simulink model "off_sentric_disc"  (R2020a)
settings: Solver=VariableStepAuto  StartTime=0.0  StopTime=10.0  RelTol=1e-3
values from neighbouring files (symbols this model uses):
  g = @(t)    [boat_riccati.m]    (also in butterfly_robot.m = [g_w;g_y_dot;g_y]; butterfly_robot_phi_varphi.m = [g_w;g_y_dot;g_y]; homework_5.m = 9.81; test_drawing.m = hgtransform)
  phi = q(2)    [butterfly_robot.m]    (also in jalla_lqr.m = atan2(y_dot,x_dot); plot_all_functions.m = linspace(0,2*pi,1000); plotting_phi_varphi.m = linspace(0,2*pi,1000); test_lmi.m = linspace(0,pi,N))
  psi = @(t) omega_c*t+psi_0    [boat_riccati.m]    (also in homework_5.m = @(x,y) (cos(y+m_g(x))^2-2)/(cos(y+m_g(x))+der_m_g(x)); jalla_lqr.m = atan2(y, x))
undefined symbols (not defined in the file or in its folder): m, mu, rcm, xcb, ycb
settings Model: Creator=g-oft  LastModifiedBy=g-oft

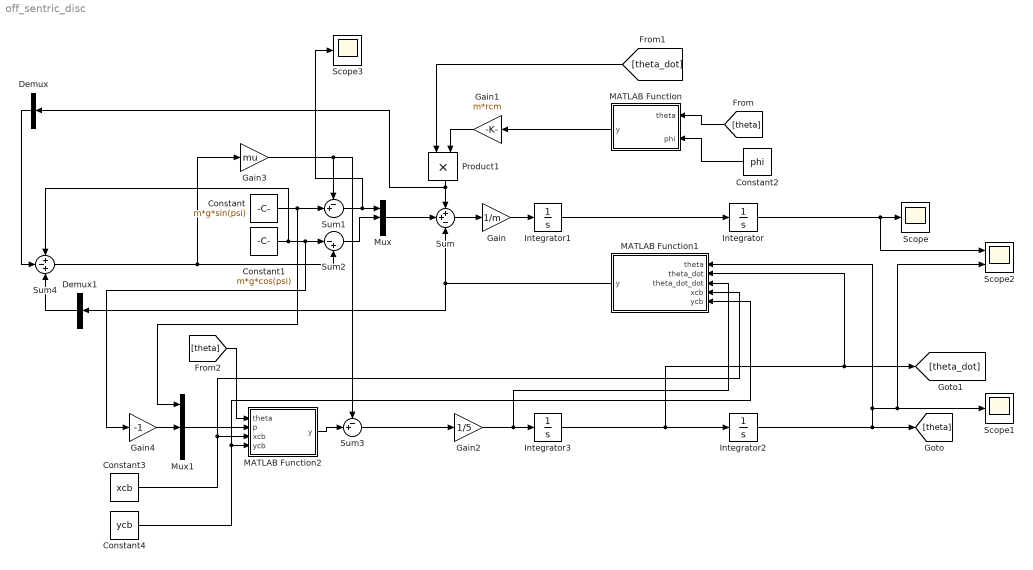
== system off_sentric_disc ==
  Constant : Constant  Value=m*g*sin(psi)
  Constant1 : Constant  Value=m*g*cos(psi)
  Constant2 : Constant  Value=phi
  Constant3 : Constant  Value=xcb
  Constant4 : Constant  Value=ycb
  Demux : Demux  Outputs=3
  Demux1 : Demux  Outputs=3
  Gain : Gain  Gain=1/m
  Gain1 : Gain  Gain=m*rcm
  Gain2 : Gain  Gain=1/5
  Gain3 : Gain  Gain=mu
  Gain4 : Gain  Gain=-1
  Integrator{,1..3} (4 alike) : Integrator
  MATLAB Function : MATLAB Function  TreatAsAtomicUnit=on
  MATLAB Function1 : MATLAB Function  TreatAsAtomicUnit=on
  MATLAB Function2 : MATLAB Function  TreatAsAtomicUnit=on
  Mux : Mux  Inputs=3
  Mux1 : Mux  Inputs=3
  Product1 : Product
  Scope : Scope
  Scope1 : Scope
  Scope2 : Scope  NumInputPorts=2
  Scope3 : Scope
  Sum : Sum  Inputs=++-
  Sum1 : Sum  Inputs=-+|
  Sum2 : Sum  Inputs=|-+
  Sum3 : Sum  Inputs=-+|
  Sum4 : Sum  Inputs=+-+
  wires:
  Integrator1/1 -> Integrator/1
  Integrator3/1 -> MATLAB Function1/2(theta_dot), [theta_dot], Integrator2/1
  Constant/1 -> Mux1/1, Sum1/2
  Sum1/1 -> Scope3/1, Mux/1
  Constant1/1 -> Gain4/1, Sum2/1, Sum4/1
  Sum2/1 -> Mux/2
  Mux/1 -> Sum/2
  Sum/1 -> Gain/1
  Gain/1 -> Integrator1/1
  [theta] -> MATLAB Function/1(theta)
  Integrator2/1 -> MATLAB Function1/1(theta), Scope2/2, Scope1/1, [theta]
  MATLAB Function/1(y) -> Gain1/1
  Product1/1 -> Demux/1, Sum/1
  Gain1/1 -> Product1/2
  [theta_dot] -> Product1/1
  Integrator/1 -> Scope2/1, Scope/1
  MATLAB Function1/1(y) -> Demux1/1, Sum/3
  Gain2/1 -> MATLAB Function1/3(theta_dot_dot), Integrator3/1
  Gain3/1 -> Sum3/1, Sum1/1
  Sum3/1 -> Gain2/1
  MATLAB Function2/1(y) -> Sum3/2
  Gain4/1 -> Mux1/2
  Mux1/1 -> MATLAB Function2/2(p)
  [theta] -> MATLAB Function2/1(theta)
  Constant3/1 -> MATLAB Function1/4(xcb), MATLAB Function2/3(xcb)
  Constant4/1 -> MATLAB Function1/5(ycb), MATLAB Function2/4(ycb)
  Constant2/1 -> MATLAB Function/2(phi)
  Demux/2 -> Sum4/2
  Demux1/2 -> Sum4/3
  Sum4/1 -> Gain3/1, Sum2/2

== matlab function off_sentric_disc/MATLAB Function1 ==
  data: theta input; y output; theta_dot input; theta_dot_dot input; xcb input; ycb input
function y = fcn(theta, theta_dot, theta_dot_dot, xcb, ycb)
a = [-cos(theta) sin(theta) 0;-sin(theta) -cos(theta) 0;0 0 1]*theta_dot^2;
b = [-sin(theta) -cos(theta) 0;cos(theta) -sin(theta) 0;0 0 1]*theta_dot_dot;
y = (a+b)*[xcb;ycb;0];

== matlab function off_sentric_disc/MATLAB Function ==
  data: theta input; y output; phi input
function y = fcn(theta, phi)
y = [cos(theta) -sin(theta) 0; sin(theta) cos(theta) 0; 0 0 1]*[cos(phi);sin(phi);0];

== matlab function off_sentric_disc/MATLAB Function2 ==
  data: theta input; y output; p input; xcb input; ycb input
function y = fcn(theta, p, xcb, ycb)
    R = [cos(theta) -sin(theta) 0;sin(theta) cos(theta) 0; 0 0 1];
    tau = R*cross([xcb;ycb;0],p);
y = tau(3);
